simulink model "sldv_speedLimiter"  (R2018b)
settings: Solver=FixedStepDiscrete  StartTime=0.0  StopTime=60  RelTol=1e-3
settings Model: Creator=jlesage  LastModifiedBy=jlesage
settings SFSimCC: SimCustomHeaderCode="#include \"speedLimiter.h\""  SimUserSources=speedLimiter.c  SimAnalyzeCustomCode=on

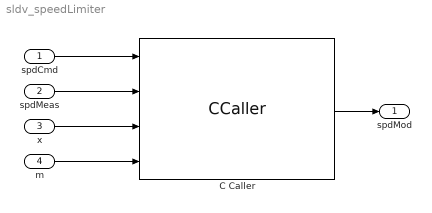
== system sldv_speedLimiter ==
  spdCmd : Inport
  spdMeas : Inport  Port=2
  x : Inport  Port=3
  m : Inport  Port=4
  C Caller : CCaller  FunctionName=speedLimiter  PortSpecificationStruct="%)30     .    T <   8    (     @         %    \"     4    !     0         %  0 \"0    $    V    07)G3F%M90  4&]R=$YA;64 4V-O<&4     26YD97@     5'EP90      4VEZ90         .    ,     8    (    !          %    \"     $    #     0         0  , ;W5T  X    X    !@    @    $          4    (     0    8    !         !     &    <W!D0VUD   .    .     8    (    !          %    \"     $    &     0         0   ...(+2311 chars)"
  spdMod : Outport
  wires:
  spdCmd/1 -> C Caller/1
  spdMeas/1 -> C Caller/2
  x/1 -> C Caller/3
  m/1 -> C Caller/4
  C Caller/1 -> spdMod/1
